simulink library "INT_EngDa_TEng"  (R2016b)
settings: Solver=VariableStepAuto  StartTime=0.0  StopTime=10.0  RelTol=1e-3
settings Model: Creator=Administrator  LastModifiedBy=Administrator

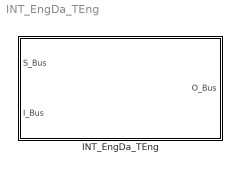
== system INT_EngDa_TEng ==
  INT_EngDa_TEng : Subsystem

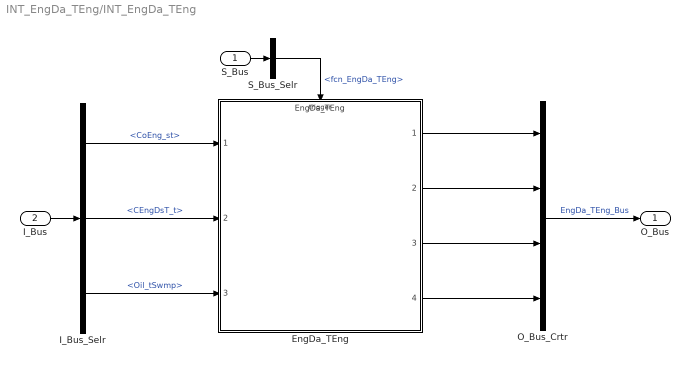
== system INT_EngDa_TEng/INT_EngDa_TEng ==
  S_Bus : Inport
  I_Bus : Inport  Port=2
  EngDa_TEng : ModelReference  ModelNameDialog=EngDa_TEng  SimulationMode=Normal  ModelReferenceVersion=1.10  TriggerPortName=function  TriggerPortTriggerType=function-call  TriggerPortStatesWhenEnabling=held
  I_Bus_Selr : BusSelector  OutputSignals=CoEng_st,CEngDsT_t,Oil_tSwmp
  O_Bus_Crtr : BusCreator  Inputs=4
  S_Bus_Selr : BusSelector  OutputSignals=fcn_EngDa_TEng
  O_Bus : Outport
  wires:
  S_Bus_Selr/1 -> EngDa_TEng/Trigger  "<fcn_EngDa_TEng>"
  S_Bus/1 -> S_Bus_Selr/1
  I_Bus/1 -> I_Bus_Selr/1
  I_Bus_Selr/1 -> EngDa_TEng/1  "<CoEng_st>"
  I_Bus_Selr/2 -> EngDa_TEng/2  "<CEngDsT_t>"
  I_Bus_Selr/3 -> EngDa_TEng/3  "<Oil_tSwmp>"
  O_Bus_Crtr/1 -> O_Bus/1  "EngDa_TEng_Bus"
  EngDa_TEng/1 -> O_Bus_Crtr/1
  EngDa_TEng/2 -> O_Bus_Crtr/2
  EngDa_TEng/3 -> O_Bus_Crtr/3
  EngDa_TEng/4 -> O_Bus_Crtr/4
